simulink model "Noa_Nofusion"  (R2020b)
settings: Solver=FixedStepDiscrete  StartTime=0.0  StopTime=Inf  FixedStep=0.01  RelTol=1e-3
PostLoadFcn:
  | if any(exist('dsrtsu_mdlpostloadfcn', 'file') ~= 0), dsrtsu_mdlpostloadfcn('Execute', bdroot); end
InitFcn:
  | , if any(exist('rtifpga_mdlclblib', 'file') ~= 0), rtifpga_mdlclblib('Init', bdroot); end,
  | , if any(exist('dsmpb_private', 'file') ~= 0), dsmpb_private('dsmpb_mdlclblib', 'Init', bdroot); end,
undefined symbols (not defined in the file or in its folder): ACC_TimeGap_DecSetSwt, ACC_TimeGap_IncSetSwt, AccelPedalPosn, AccelPedalPosnVldty, AccelPedlPosnDiagc, AccPedalOverride, ACU_ShiftInProgress, ADAS_Posn_CurLane, AESSwtReq, ALC_SwtReq, BrkPedalSts, CC_ACC_CANCEL_OFFSwt, CC_ACC_CRUISE_OFFSwt, CC_ACC_DecSetSpd_SetSwt, CC_ACC_IncSetSpd_ResuSwt, CC_ACCSwtErr, CharSpd_ms, CSA_NODE, CURRENT_GEAR, CurrentGearValid, DiscIntNeverNeededParam, DrvDoorSts, DrvSBR, DrvTrqReqOvld, ECMACCInterface, ECMRespACC, ELKSwtReq, EngLimpHomeSts, EngSpd, EngState, EngState_PHEV, EngTrqMaxActSpd, EngTrqMinAct, EPS_DrvInpTrqVal_HighReslolution, EPS_FailSts, EPS_LKATorqOvrlDlvd, EPS_LKATorqOvrlDlvdVld, EPS_LKATrqOvlDlvdSts, EPS_SteerMod, EPS_TrqSnsrSts, EQ4_APPINFO, EQ4_LA_ELEM, EQ4_LA_HDR, EQ4_LAP_ELEM, EQ4_LAP_HDR, EQ4_LH_ELEM, EQ4_LH_HDR, EQ4_LRE_ELEM, EQ4_LRE_HDR, ESS_PedSwtReq, ESS_VehSwtReq, FFogLmpSts_F_Pbox, FLWheelDriveDirection, FLWheelSpd, FrntWiprSwtSts, FrntWshrSwtSts, FRWheelDriveDirection, FRWheelSpd, HazardLmpSwtSts, HCU_AccelPedalPosn_Diag ... (+151)
libraries: simulink x144, dsmpblib x33, canfdmsglib x10
(part 19 of 20)

== matlab function Noa_Nofusion/TOS/Subsystem2/DOP/HWA_Task100ms1/Dyc ==
  data: kapTrajFiltK1 input single size=1; vRef input single size=1; kapTrajFilt output single size=1; kapCourseErr output single; kapTraj input single size=1; alpSideSlipAngle input single size=1; A2 input single size=1; A1 input single size=1; LineValid input boolean size=1; ObjDx input single size=15; ObjDy input single size=15; TarLineValid input boolean; TarLineA2 input single; TarLineA1 input single; TarLineA0 input single size=1; dxC0 output single size=1; aPC0 output single size=1; bPC0 output single size=1; cPC0 output single size=1; aPC1 output single size=1; bPC1 output single size=1; cPC1 output single size=1; ObjDyc output single size=15
function [kapTrajFilt,kapCourseErr,dxC0,aPC0,bPC0,cPC0,aPC1,bPC1,cPC1,ObjDyc] = ...
    DriveCourseCalc(kapTrajFiltK1,vRef,kapTraj,alpSideSlipAngle,...
    A2,A1,LineValid,ObjDx,ObjDy,TarLineValid,TarLineA2,TarLineA1,TarLineA0)

ObjDyc = single(zeros(15,1));

if vRef>8.33
    t_alpSideSlipAngle = -alpSideSlipAngle;
else
    t_alpSideSlipAngle = single(0);
end

temp1 = single(0.1)/(single(0.1) + interpolate(single(24),single(0),single(55),single(0.4),vRef));

kapTrajFilt = kapTrajFiltK1 + temp1*(kapTraj - kapTrajFiltK1);

temp1 = abs(kapTraj*vRef);

if (temp1<0.001)&&(vRef>8.3)
    t_kapTrajwHyst = single(0);
else
    t_kapTrajwHyst = kapTrajFilt;
end

if TarLineValid
    temp = interpolate(single(0.2),single(0.2),single(1.5),single(1),abs(TarLineA0));
    dxC0Min = single(3);
else
    temp = single(1);
    dxC0Min = single(10);
end

dxC0 = max(vRef*temp,dxC0Min);
aPC0 = 0.5*t_kapTrajwHyst*(single(1)+1.5*t_alpSideSlipAngle*t_alpSideSlipAngle);
bPC0 = t_alpSideSlipAngle;
cPC0 = single(0);

temp1 = single(0.1)*abs(t_kapTrajwHyst);
temp2 = min(single(0.00013),single(0.004)/max(vRef,single(10)));
kapCourseErr = max(temp1,temp2);

aPC1 = aPC0;
bPC1 = bPC0;
cPC1 = single(0);

Low = interpolate(single(4),single(1),single(20),single(0),abs(atan(A1)));    % low vehiclespeed lanechange Angle is 4deg~20deg;
High = interpolate(single(4),single(1),single(10),single(0),abs(atan(A1)));   % low vehiclespeed lanechange Angle is 4deg~10deg;
t_vRefFactor = interpolate(single(5),Low,single(25),High,vRef);

t_Factor = single(1)*t_vRefFactor;

if TarLineValid==true
    aPC1 = TarLineA2;
    bPC1 = TarLineA1;
    cPC1 = (aPC0 - aPC1)*dxC0*dxC0 + (bPC0 - bPC1)*dxC0;
else
    if LineValid
        aPC1 = aPC0*(1 - t_Factor) + A2*t_Factor;
        bPC1 = bPC0*(1 - t_Factor) + A1*t_Factor;
        cPC1 = (aPC0 - aPC1)*dxC0*dxC0 + (bPC0 - bPC1)*dxC0;
    end
end

for i=1:15
   if ObjDx(i)>dxC0
      ObjDyc(i) =  ObjDy(i) - (aPC1*ObjDx(i)*ObjDx(i) + bPC1*ObjDx(i) + cPC1);
   else
      ObjDyc(i) =  ObjDy(i) - (aPC0*ObjDx(i)*ObjDx(i) + bPC0*ObjDx(i));
   end
end
end


function out = interpolate(x1,z1,x2,z2,Raw)
if Raw<=x1
    out = z1;
else
    if Raw>=x2
        out = z2;
    else
        out = z1 + (Raw-x1)*(z2-z1)/(x2-x1);
    end
end
end

== matlab function Noa_Nofusion/CR_RSDS_Input/MATLAB Function1 ==
  data: ObjNumber input uint8 size=1; ObjPrio output single size=24; ObjID input uint8 size=24; ObjDx input single size=24; ObjMatrix output single size=24
function [ObjPrio,ObjMatrix] = fcn(ObjNumber,ObjID,ObjDx)
%#codegen
ObjPrio = single(zeros(24,1));

for i=1:ObjNumber
    if ObjID(i)>0
        ObjPrio(i)=single(255) - abs(ObjDx(i));
    else
        ObjPrio(i)=single(0);
    end
end

ObjMatrix=ObjPrio;

t_h=1;
while 1
    t_h = t_h*3+1;
    if t_h>=ObjNumber
        break;
    end
end

%   t_h = 121;
while 1
    t_h = fix(t_h/3);
    for i=(t_h+1):ObjNumber
        j=i;
        t_zw=ObjMatrix(i);
        while (j>t_h)&&(t_zw<ObjMatrix(j-t_h))
            ObjMatrix(j)=ObjMatrix(j-t_h);
            j=j-t_h;
        end
        ObjMatrix(j)=t_zw;
    end
    if t_h==1
        break;
    end
end
end

== matlab function Noa_Nofusion/CR_RSDS_Input/MATLAB Function2 ==
  data: Prio input single size=24; Matrix input single size=24; ID input uint8 size=24; ObjID output uint8 size=11; Dx input single size=24; Dy input single size=24; ObjDx output single size=11; Vx input single size=24; Vy input single size=24; Ax input single size=24; Age input uint8 size=24; MoveSts input uint8 size=24; ObjDy output single size=11; ObjVx output single size=11; ObjVy output single size=11; ObjAx output single size=11; ObjAge output uint8 size=11; ObjMoveSts output uint8 size=11; FusType input uint8 size=24; ObjFusType output uint8 size=11
function [ObjID,ObjDx,ObjDy,ObjVx,ObjVy,ObjAx,ObjAge,ObjMoveSts,ObjFusType] =...
    fcn(Prio,Matrix,ID,Dx,Dy,Vx,Vy,Ax,Age,MoveSts,FusType)
%#codegen
ObjPrioLimit = Matrix(24-11);
ObjID = uint8(zeros(11,1));
ObjDx = single(zeros(11,1));
ObjDy = single(zeros(11,1));
ObjVx = single(zeros(11,1));
ObjVy = single(zeros(11,1));
ObjAx = single(zeros(11,1));
ObjAge = uint8(zeros(11,1));
ObjMoveSts = uint8(zeros(11,1));
ObjFusType = uint8(zeros(11,1));
Num = uint8(0);

for i=1:24
  if ID(i)>0 && Prio(i)>ObjPrioLimit
      Num = Num + uint8(1);
      ObjID(Num) = uint8(i);
      ObjDx(Num) = Dx(i);
      ObjDy(Num) = Dy(i);
      ObjVx(Num) = Vx(i);
      ObjVy(Num) = Vy(i);
      ObjAx(Num) = Ax(i);
      ObjAge(Num) = Age(i);
      ObjMoveSts(Num) = MoveSts(i);
      ObjFusType(Num) = FusType(i);
  end
end

== matlab function Noa_Nofusion/CR_RSDS_Input/RSDS_L_Bus/RSDS_L ==
  data: RadarID input uint8 size=1; ID input uint8 size=6; Dx input single size=6; Dy input single size=6; Vx input single size=6; Vy input single size=6; Ax input single size=6; ObjIDK1 input uint8 size=6; P output uint8 size=6; ObjDx output single size=6; ObjDy output single size=6; ObjVx output single size=6; ObjVy output single size=6; ObjAx output single size=6; ObjMoveSts output uint8 size=6; ObjFusType output uint8 size=6; ObjID output uint8 size=6; ObjAgeK1 input uint8 size=6; ObjAge output uint8 size=6
function [P,ObjDx,ObjDy,ObjVx,ObjVy,ObjAx,ObjMoveSts,ObjFusType,ObjID,ObjAge] =...
    DataT(RadarID,ID,Dx,Dy,Vx,Vy,Ax,ObjIDK1,ObjAgeK1)

if RadarID==uint8(1)
    FusFac = 4;
elseif RadarID==uint8(2)
    FusFac = 8;
elseif RadarID==uint8(3)
    FusFac = 16;
else
    FusFac = 32;
end

ObjID = uint8(zeros(6,1));
ObjDx = single(zeros(6,1));
ObjDy = single(zeros(6,1));
ObjVx = single(zeros(6,1));
ObjVy = single(zeros(6,1));
ObjAx = single(zeros(6,1));
ObjAge = uint8(ones(6,1));
ObjMoveSts = uint8(2*ones(6,1));
ObjFusType = uint8(FusFac*ones(6,1));

T = uint8(zeros(6,1));
P = uint8(zeros(6,1));
Index01 = uint8(zeros(6,1));
Index02 = uint8(zeros(6,1));
M = uint8(0);
N = uint8(0);
w = uint8(0);

for i=uint8(1):uint8(6)
    for j=uint8(1):uint8(6)
        if ID(i)==ObjIDK1(j) && ID(i)>uint8(0)
            T(j) = i;
            P(i) = j;
        end
    end
end

for j=uint8(1):uint8(6)
    if T(j)==uint8(0)
        if ObjIDK1(j)==uint8(0)
            N = N + uint8(1);
            Index01(N) = j;
        else
            M = M + uint8(1);
            Index02(M) = j;
        end
    end
end

for i=uint8(1):uint8(6)
    if P(i)==uint8(0) && ID(i)>uint8(0)
        w = w + uint8(1);
        if w<=N
            P(i) = Index01(w);
        else
            P(i) = Index02(w - N);
        end
    elseif P(i)>uint8(0)
        ObjAge(P(i)) = min(ObjAgeK1(i) + uint8(1),uint8(255));
    end
    if P(i)>uint8(0)
       ObjID(P(i)) = ID(i);
       ObjDx(P(i)) = Dx(i);
       ObjDy(P(i)) = Dy(i);
       ObjVx(P(i)) = Vx(i);
       ObjVy(P(i)) = Vy(i);
       ObjAx(P(i)) = Ax(i);
    end
end
for i=uint8(1):uint8(6)
    if ObjID(i)==uint8(0)
        ObjAge(i) = uint8(0);
        ObjMoveSts(i) = uint8(0);
        ObjFusType(i) = uint8(0);
    end
end
end

== matlab function Noa_Nofusion/CR_RSDS_Input/RSDS_R_Bus/RSDS_R ==
  data: RadarID input uint8 size=1; ID input uint8 size=6; Dx input single size=6; Dy input single size=6; Vx input single size=6; Vy input single size=6; Ax input single size=6; ObjIDK1 input uint8 size=6; P output uint8 size=6; ObjDx output single size=6; ObjDy output single size=6; ObjVx output single size=6; ObjVy output single size=6; ObjAx output single size=6; ObjMoveSts output uint8 size=6; ObjFusType output uint8 size=6; ObjID output uint8 size=6; ObjAgeK1 input uint8 size=6; ObjAge output uint8 size=6
function [P,ObjDx,ObjDy,ObjVx,ObjVy,ObjAx,ObjMoveSts,ObjFusType,ObjID,ObjAge] =...
    DataT(RadarID,ID,Dx,Dy,Vx,Vy,Ax,ObjIDK1,ObjAgeK1)

if RadarID==uint8(1)
    FusFac = 4;
elseif RadarID==uint8(2)
    FusFac = 8;
elseif RadarID==uint8(3)
    FusFac = 16;
else
    FusFac = 32;
end

ObjID = uint8(zeros(6,1));
ObjDx = single(zeros(6,1));
ObjDy = single(zeros(6,1));
ObjVx = single(zeros(6,1));
ObjVy = single(zeros(6,1));
ObjAx = single(zeros(6,1));
ObjAge = uint8(ones(6,1));
ObjMoveSts = uint8(2*ones(6,1));
ObjFusType = uint8(FusFac*ones(6,1));

T = uint8(zeros(6,1));
P = uint8(zeros(6,1));
Index01 = uint8(zeros(6,1));
Index02 = uint8(zeros(6,1));
M = uint8(0);
N = uint8(0);
w = uint8(0);

for i=uint8(1):uint8(6)
    for j=uint8(1):uint8(6)
        if ID(i)==ObjIDK1(j) && ID(i)>uint8(0)
            T(j) = i;
            P(i) = j;
        end
    end
end

for j=uint8(1):uint8(6)
    if T(j)==uint8(0)
        if ObjIDK1(j)==uint8(0)
            N = N + uint8(1);
            Index01(N) = j;
        else
            M = M + uint8(1);
            Index02(M) = j;
        end
    end
end

for i=uint8(1):uint8(6)
    if P(i)==uint8(0) && ID(i)>uint8(0)
        w = w + uint8(1);
        if w<=N
            P(i) = Index01(w);
        else
            P(i) = Index02(w - N);
        end
    elseif P(i)>uint8(0)
        ObjAge(P(i)) = min(ObjAgeK1(i) + uint8(1),uint8(255));
    end
    if P(i)>uint8(0)
       ObjID(P(i)) = ID(i);
       ObjDx(P(i)) = Dx(i);
       ObjDy(P(i)) = Dy(i);
       ObjVx(P(i)) = Vx(i);
       ObjVy(P(i)) = Vy(i);
       ObjAx(P(i)) = Ax(i);
    end
end
for i=uint8(1):uint8(6)
    if ObjID(i)==uint8(0)
        ObjAge(i) = uint8(0);
        ObjMoveSts(i) = uint8(0);
        ObjFusType(i) = uint8(0);
    end
end
end

== matlab function Noa_Nofusion/TOS/Subsystem2/DOP/HWA_Task100ms1/DycCutIn ==
  data: ObjValid input boolean size=15; ObjDyc input single size=15; ObjMoveSts input uint8 size=15; ObjDycCutIn output single size=15; ObjMove_b output boolean size=15; ObjCnt input uint8 size=15; ObjDycHist input single size=15; ObjqDycHist input single size=15; dycFiltK1 input single size=15; ObjDycFilt output single size=15
function [ObjDycCutIn,ObjMove_b,ObjDycFilt] = ...
    ObjDycCutInCalc(ObjValid,ObjDyc,ObjMoveSts,ObjCnt,ObjDycHist,ObjqDycHist,dycFiltK1)
 
ObjDycCutIn = single(zeros(15,1));
ObjDycFilt = single(zeros(15,1));
ObjMove_b = false(15,1); 
 
for i=1:15
    if ObjValid(i)
        t_dyc = ObjDyc(i);
        t_dycHist = ObjDycHist(i);
        t_qDycHist = ObjqDycHist(i);
        
        weightDycHist = t_qDycHist*0.1;
        weightDyc = single(1) - weightDycHist;
        
        t_dycASI = weightDycHist*t_dycHist + weightDyc*t_dyc;
        ObjDycCutIn(i) = t_dycASI;
        
        if ObjCnt(i)>2
            ObjDycFilt(i) = 0.028*(t_dycASI - dycFiltK1(i)) + dycFiltK1(i);
        else
            ObjDycFilt(i) = t_dycASI;
        end
        if ObjMoveSts(i)==2
            ObjMove_b(i) = true;
        end
    end
end

== matlab function Noa_Nofusion/SimBCM/BCMsim ==
  data: SimLeLmp input; CSASim_LampReq output; SimRiLmp input; Model_IDC_L2_LampReq input
function CSASim_LampReq = fcn(SimLeLmp, SimRiLmp, Model_IDC_L2_LampReq)
CSASim_LampReq=Model_IDC_L2_LampReq;
if SimRiLmp
    CSASim_LampReq=uint8(2);
end
if SimLeLmp
    CSASim_LampReq=uint8(1);
end

== matlab function Noa_Nofusion/TOS/Subsystem2/DOP/HWA_Task100ms1/DycHistCalc ==
  data: TrajHistBufferBTrajEnd input boolean; ObjTrajNumber input uint8; ObjDycHist output single; TrajCurrentIndex input uint8; TrajHistBufferBValid input boolean; TrajHistBufferDxv input single; TrajHistBufferDyv input single; ObjValid input boolean; ObjqDycHist output single; dxC0 input; aP0 input; bP0 input; cP0 input; aP1 input; bP1 input; cP1 input
function [ObjDycHist,ObjqDycHist] = DycHistCalc(TrajHistBufferBTrajEnd,ObjTrajNumber,TrajCurrentIndex,...
    TrajHistBufferBValid,TrajHistBufferDxv,TrajHistBufferDyv,ObjValid,dxC0,aP0,bP0,cP0,aP1,bP1,cP1)

t_dxv = single(0);
t_dyv = single(0);
t_dxvK1 = single(0);
t_dyvK1 = single(0);
ObjDycHist = single(zeros(15,1));
ObjqDycHist = single(zeros(15,1));

for iObj=1:15
    t_TrajNumber = ObjTrajNumber(iObj);
    if t_TrajNumber<21
        t_End = false;
        t_Failed = false;
        t_TrajCurrentIndex = TrajCurrentIndex(t_TrajNumber);
        t_TrajEnd = TrajHistBufferBTrajEnd(t_TrajNumber,t_TrajCurrentIndex);
        if (ObjValid(iObj)==true)&&(t_TrajEnd==false)
            for k=1:24
                if t_End==false
                    if t_TrajCurrentIndex<k
                        t_Index = t_TrajCurrentIndex + uint8(25) - k;
                    else
                        t_Index = t_TrajCurrentIndex - k + uint8(1);
                    end
                    if t_Index==1
                        t_IndexK1 = uint8(24);
                    else
                        t_IndexK1 = t_Index - uint8(1);
                    end
                    t_ValidK1 = TrajHistBufferBValid(t_TrajNumber,t_IndexK1);
                    t_TrajEndK1 = TrajHistBufferBTrajEnd(t_TrajNumber,t_IndexK1);
                    t_dxv = TrajHistBufferDxv(t_TrajNumber,t_Index);
                    t_dxvK1 = TrajHistBufferDxv(t_TrajNumber,t_IndexK1);
                    t_dyv = TrajHistBufferDyv(t_TrajNumber,t_Index);
                    t_dyvK1 = TrajHistBufferDyv(t_TrajNumber,t_IndexK1);
                    
                    if (t_TrajEndK1==true)||(t_ValidK1==false)
                        t_End = true;
                        t_Failed = true;
                    end
                    if (t_dxv>=0)&&(t_dxvK1<=0)
                        t_End = true;
                    end
                end
            end
        end
        if (t_End==true)&&(t_Failed==false)
            if (t_dxv==t_dxvK1)
                t_dycHist = t_dyv;
            else
                t_dycHist = t_dyv - t_dxv*(t_dyvK1 - t_dyv)/(t_dxvK1 - t_dxv);
            end
            t_qDycHist = single(1);  
        else
            if (t_End==true)&&(t_Failed==true)&&(t_dxv>0)
                if t_dxv>(dxC0)
                    t_dycHist = t_dyv - (aP1*t_dxv*t_dxv + bP1*t_dxv + cP1); 
                else
                    t_dycHist = t_dyv - (aP0*t_dxv*t_dxv + bP0*t_dxv + cP0); 
                end
               t_qDycHist = max((single(80) - t_dxv)/single(80),single(0));
            else
                t_dycHist = single(0);
                t_qDycHist = single(0);
            end
        end
    else
        t_dycHist = single(0);
        t_qDycHist = single(0);
    end
    ObjDycHist(iObj) = t_dycHist;
    ObjqDycHist(iObj) = t_qDycHist;
end

== stateflow chart Noa_Nofusion/SimBCM/CSALampCtrlSim/Chart1 ==
  state OFF
    en:
    SwtSts=false;
  state Hold
    en:
    SwtSts=true;
  state LeCloseReady
  (default) -> OFF
  LeCloseReady -> OFF : [SteerWheelAng<P_LmpCloseAngClose...
      | ||OFF]
  Hold -> OFF [order 2] : [OFF]
  OFF -> Hold : [ON]
  Hold -> LeCloseReady [order 1] : [SteerWheelAng>P_LmpCloseAngReady]
  data: SwtSts output; OFF input; ON input; SteerWheelAng input; P_LmpCloseAngClose input; P_LmpCloseAngReady input

== matlab function Noa_Nofusion/Subsystem4/LHLine ==
  data: LH_Count input; LH1A0 input single size=1; LH1A1 input single size=1; LH1A2 input single size=1; LH1A3 input single size=1; LH1RaMin input single size=1; LH1RaMax input single size=1; LH1Conf output uint8 size=1; LH1Avail input uint8 size=1; LH1LineType input uint8 size=1; LH1DLType input uint8 size=1; LH1SideType input uint8 size=1; LH1Wid input single size=1; LH1Crossing input; LH1Confidence input; LH2A0 input single size=1; LH2A1 input single size=1; LH2A2 input single size=1; LH2A3 input single size=1; LH2RaMin input single size=1; LH2RaMax input single size=1; LH2Avail input uint8 size=1; LH2LineType input uint8 size=1; LH2DLType input uint8 size=1; LH2SideType input uint8 size=1; LH2Wid input single size=1; LH1C0 output single size=1; LH1C1 output single size=1; LH1C2 output single size=1; LH1C3 output single size=1; LH1DxMin output single size=1; LH1DxMax output single size=1; LH1Type output uint8 size=1; LH1DLM output uint8 size=1; LH1Width output single size=1; LH1Reliable output; LeftLaneChange output uint8 size=1; LH2Conf output uint8 size=1; LH2C0 output single size=1; LH2C1 output single size=1; LH2C2 output single size=1; LH2C3 output single size=1; LH2DxMin output single size=1; LH2DxMax output single size=1; LH2Type output uint8 size=1; LH2DLM output uint8 size=1; LH2Width output single size=1; LH2Reliable output; RightLaneChange output uint8 size=1; LH2Crossing input; LH2Confidence input
function [LH1Conf,LH1C0,LH1C1,LH1C2,LH1C3,LH1DxMin,LH1DxMax,LH1Type,LH1DLM,LH1Width,LH1Reliable,LeftLaneChange,...
    LH2Conf,LH2C0,LH2C1,LH2C2,LH2C3,LH2DxMin,LH2DxMax,LH2Type,LH2DLM,LH2Width,LH2Reliable,RightLaneChange]...
    = LH(LH_Count,LH1A0,LH1A1,LH1A2,LH1A3,LH1RaMin,LH1RaMax,LH1Avail,LH1LineType,LH1DLType,LH1SideType,LH1Wid,LH1Crossing,LH1Confidence,...
    LH2A0,LH2A1,LH2A2,LH2A3,LH2RaMin,LH2RaMax,LH2Avail,LH2LineType,LH2DLType,LH2SideType,LH2Wid,LH2Crossing,LH2Confidence)

LH1Conf = uint8(0);
LH1C0 = single(0);
LH1C1 = single(0);
LH1C2 = single(0);
LH1C3 = single(0);
LH1DxMin = single(0);
LH1DxMax = single(0);
LH1Type = uint8(0);
LH1DLM = uint8(0);
LH1Width = single(0);
LH1Reliable = single(0);
LeftLaneChange = uint8(0);

LH2Conf = uint8(0);
LH2C0 = single(0);
LH2C1 = single(0);
LH2C2 = single(0);
LH2C3 = single(0);
LH2DxMin = single(0);
LH2DxMax = single(0);
LH2Type = uint8(0);
LH2DLM = uint8(0);
LH2Width = single(0);
LH2Reliable = single(0);
RightLaneChange = uint8(0);


%%
if LH_Count >= 1
    if LH1SideType==1
        LH1Conf = LH1Avail;
        LH1C0 = LH1A0;
        LH1C1 = LH1A1;
        LH1C2 = LH1A2;
        LH1C3 = LH1A3;
        LH1DxMin = LH1RaMin;
        LH1DxMax = LH1RaMax;
        LH1Type = LH1LineType;
        LH1DLM = LH1DLType;
        LH1Width = LH1Wid;
        LH1Reliable = LH1Confidence;
        LeftLaneChange = LH1Crossing;
    elseif LH1SideType==2
        LH2Conf = LH1Avail;
        LH2C0 = LH1A0;
        LH2C1 = LH1A1;
        LH2C2 = LH1A2;
        LH2C3 = LH1A3;
        LH2DxMin = LH1RaMin;
        LH2DxMax = LH1RaMax;
        LH2Type = LH1LineType;
        LH2DLM = LH1DLType;
        LH2Width = LH1Wid;
        LH2Reliable = LH1Confidence;
        RightLaneChange = LH1Crossing;
    end
    if LH_Count >= 2
        if LH2SideType==1
            LH1Conf = LH2Avail;
            LH1C0 = LH2A0;
            LH1C1 = LH2A1;
            LH1C2 = LH2A2;
            LH1C3 = LH2A3;
            LH1DxMin = LH2RaMin;
            LH1DxMax = LH2RaMax;
            LH1Type = LH2LineType;
            LH1DLM = LH2DLType;
            LH1Width = LH2Wid;
            LH1Reliable = LH2Confidence;
            LeftLaneChange = LH2Crossing;
        elseif LH2SideType==2
            LH2Conf = LH2Avail;
            LH2C0 = LH2A0;
            LH2C1 = LH2A1;
            LH2C2 = LH2A2;
            LH2C3 = LH2A3;
            LH2DxMin = LH2RaMin;
            LH2DxMax = LH2RaMax;
            LH2Type = LH2LineType;
            LH2DLM = LH2DLType;
            LH2Width = LH2Wid;
            LH2Reliable = LH2Confidence;
            RightLaneChange = LH2Crossing;
        end
    end
end

== matlab function Noa_Nofusion/Subsystem4/MATLAB Function5 ==
  data: IFV2RearAxis input single size=1; a0 output single size=1; a1 output single size=1; a2 output single size=1; a3 output single size=1; IFV2CenterAxis input single size=1; A0 input single size=1; A1 input single size=1; A2 input single size=1; A3 input single size=1; Range_min input single size=1; Rmin output single size=1; Range_max input single size=1; Rmax output single size=1
function [a0,a1,a2,a3,Rmin,Rmax] = ...
    fcn(IFV2RearAxis,IFV2CenterAxis,A0,A1,A2,A3,Range_min,Range_max)

Rmin = Range_min + IFV2RearAxis;
Rmax = Range_max + IFV2RearAxis;

if Range_max>0
   xi = [10;20;40;80];
   yi = -A3*xi.^3 - A2*xi.^2 - A1*xi - A0 + IFV2CenterAxis;
   xi = xi + IFV2RearAxis;
   [a3,a2,a1,a0] = pl(xi,yi);
else
    a3 = single(0);
    a2 = single(0);
    a1 = single(0);
    a0 = single(0);
end

== matlab function Noa_Nofusion/Subsystem4/MATLAB Function6 ==
  data: IFV2RearAxis input single size=1; a0 output single size=1; a1 output single size=1; a2 output single size=1; a3 output single size=1; IFV2CenterAxis input single size=1; A0 input single size=1; A1 input single size=1; A2 input single size=1; A3 input single size=1; Range_min input single size=1; Rmin output single size=1; Range_max input single size=1; Rmax output single size=1
function [a0,a1,a2,a3,Rmin,Rmax] = ...
    fcn(IFV2RearAxis,IFV2CenterAxis,A0,A1,A2,A3,Range_min,Range_max)

Rmin = Range_min + IFV2RearAxis;
Rmax = Range_max + IFV2RearAxis;

if Range_max>0
   xi = [10;20;40;80];
   yi = -A3*xi.^3 - A2*xi.^2 - A1*xi - A0 + IFV2CenterAxis;
   xi = xi + IFV2RearAxis;
   [a3,a2,a1,a0] = pl(xi,yi);
else
    a3 = single(0);
    a2 = single(0);
    a1 = single(0);
    a0 = single(0);
end

== matlab function Noa_Nofusion/Subsystem4/Simulink Function/MATLAB Function3 ==
  data: IFV2RearAxis input single size=1; a0 output single size=1; a1 output single size=1; a2 output single size=1; a3 output single size=1; IFV2CenterAxis input single size=1; A0 input single size=1; A1 input single size=1; A2 input single size=1; A3 input single size=1; Range_min input single size=1; Rmin output single size=1; Range_max input single size=1; Rmax output single size=1
function [a0,a1,a2,a3,Rmin,Rmax] = ...
    fcn(IFV2RearAxis,IFV2CenterAxis,A0,A1,A2,A3,Range_min,Range_max)

Rmin = Range_min + IFV2RearAxis;
Rmax = Range_max + IFV2RearAxis;

if Range_max>0
   xi = [10;20;40;80];
   yi = -A3*xi.^3 - A2*xi.^2 - A1*xi - A0 + IFV2CenterAxis;
   xi = xi + IFV2RearAxis;
   [a3,a2,a1,a0] = pl(xi,yi);
else
    a3 = single(0);
    a2 = single(0);
    a1 = single(0);
    a0 = single(0);
end

== stateflow chart Noa_Nofusion/SimBCM/CSALampCtrlSim/Chart2 ==
  state OFF
    en:
    SwtSts=false;
  state Hold
    en:
    SwtSts=true;
  state LeCloseReady
  (default) -> OFF
  LeCloseReady -> OFF : [abs(SteerWheelAng)>-P_LmpCloseAngClose...
      | ||OFF]
  Hold -> OFF [order 2] : [OFF]
  OFF -> Hold : [ON]
  Hold -> LeCloseReady [order 1] : [SteerWheelAng<-P_LmpCloseAngReady]
  data: SwtSts output; OFF input; ON input; SteerWheelAng input; P_LmpCloseAngClose input; P_LmpCloseAngReady input

== matlab function Noa_Nofusion/TOS/Subsystem2/DOP/HWA_Task100ms1/LostTargetCalc ==
  data: ObjValid input boolean size=15; ReID output uint8 size=1; ObjDx input single size=15; ObjDy input single size=15; DeltaDx input single size=1; DeltaDy input single size=1; P0IDK1 input uint8 size=1; P0VxK1 input single size=1; P0DxK1 input single size=1; P0DyK1 input single size=1; P0RangeK1 input; P0ArGK1 input; P0DycK1 input single size=1; P0VycK1 input single size=1; P0CutIn_bK1 input boolean size=1; tTargetLostK1 input single size=1; ReRange output single size=1; ReArG output single size=1; ReDx output single size=1; ReDy output single size=1; ReVx output single size=1; ReCutIn_b output boolean size=1; ReDyc output single size=1; ReVyc output single size=1; TargetLost_b output boolean size=1; Covered_b output boolean size=1; tTargetLost output single size=1
function [ReID,ReRange,ReArG,ReDx,ReDy,ReVx,ReCutIn_b,ReDyc,ReVyc,TargetLost_b,Covered_b,tTargetLost]...
    = LostTargetCalc(ObjValid,ObjDx,ObjDy,DeltaDx,DeltaDy,...
    P0IDK1,P0VxK1,P0DxK1,P0DyK1,P0RangeK1,P0ArGK1,P0DycK1,P0VycK1,P0CutIn_bK1,tTargetLostK1)
 
ReID = P0IDK1;
ReRange = single(255);
ReArG = single(0);
ReDx = single(255);
ReDy = single(0);
ReVx = single(0);
ReDyc = single(0);
ReVyc = single(0);
ReCutIn_b = false;
TargetLost_b = false;
tTargetLost = single(0);
Covered_b = false;
 
if (P0IDK1>0)&&(P0IDK1<100)    % k1 Exist Target
    if ObjValid(P0IDK1)==false
        ExistNearObj = false;
        P0DxPred = P0DxK1 + 0.1*P0VxK1;
        P0DyPred = P0DyK1;
        P0RangePred = P0RangeK1 + 0.1*P0VxK1; 
        for i=1:15
            if (ObjValid(i)==true)&&(ObjDx(i)<P0DxPred)
                Covered_b = CoveredCalc(P0DxPred,P0DyPred,ObjDx(i),ObjDy(i),single(2.1),single(-0.1));
                if Covered_b==true
                   break; 
                end
            end
            if (ObjValid(i)==1)&&(abs(ObjDx(i)-P0DxPred)<DeltaDx)&&(abs(ObjDy(i)-P0DyPred)<DeltaDy)
               ExistNearObj = true;
               ReID = uint8(i);
               ReDx = ObjDx(i);
            end
        end
        if (ExistNearObj==false)&&(Covered_b==false)
            TargetLost_b = true;
            tTargetLost = single(0.1);
            ReID = uint8(255);
            ReRange = P0RangePred;
            ReArG = P0ArGK1;
            ReDx = P0DxPred;
            ReDy = P0DyPred;
            ReVx = P0VxK1;
            ReCutIn_b = P0CutIn_bK1;
            ReVyc = P0VycK1;
            ReDyc = P0DycK1 + 0.1*P0VycK1;
        end
    end
else
    if P0IDK1>100   %  k1 Exist Target Re
        ExistNearObj = false;
        P0DxPred = P0DxK1 + 0.1*P0VxK1;
        P0DyPred = P0DyK1;
        P0RangePred = P0RangeK1 + 0.1*P0VxK1; 

        for i=1:15
            if (ObjValid(i)==1)&&(abs(ObjDx(i)-P0DxPred)<DeltaDx)&&(abs(ObjDy(i)-P0DyPred)<DeltaDy)
                ExistNearObj = true;
                ReID = uint8(i);
                ReDx = ObjDx(i);
                TargetLost_b = false;
                tTargetLost = single(0);
            end
        end
        if ExistNearObj==false
            TargetLost_b = true;
            tTargetLost = tTargetLostK1 + single(0.1);
            ReID = uint8(255);
            ReRange = P0RangePred;
            ReArG = P0ArGK1;
            ReDx = P0DxPred;
            ReDy = P0DyPred;
            ReVx = P0VxK1;
            ReCutIn_b = P0CutIn_bK1;
            ReVyc = P0VycK1;
            ReDyc = P0DycK1 + 0.1*P0VycK1;
        end
    end
end
end
 
function t_Covered_b = CoveredCalc(DxPred,DyPred,Dx,Dy,IFVDx,IFVDy)
y = (IFVDy - DyPred)*(Dx - DxPred)/(IFVDx - DxPred) + DyPred ;
Delta = single(0.8) + (Dx - IFVDx)/(DxPred - IFVDx);
if abs(Dy - y)<=Delta
    t_Covered_b = true;
else
    t_Covered_b = false;
end
end

== matlab function Noa_Nofusion/Subsystem4/LALine ==
  data: LA_Count input; L1Conf output uint8 size=1; L1C0 output single size=1; L1C1 output single size=1; L1C2 output single size=1; L1C3 output single size=1; L1DxMin output single size=1; L1DxMax output single size=1; L1A0 input single size=1; L1A1 input single size=1; L1A2 input single size=1; L1A3 input single size=1; L1RaMin input single size=1; L1RaMax input single size=1; L1Avail input uint8 size=1; L1LineType input uint8 size=1; L1DLType input uint8 size=1; L1SideType input uint8 size=1; L1Wid input single size=1; L1Confidence input; L2A0 input single size=1; L2A1 input single size=1; L2A2 input single size=1; L2A3 input single size=1; L2RaMin input single size=1; L2RaMax input single size=1; L2Avail input uint8 size=1; L2LineType input uint8 size=1; L2DLType input uint8 size=1; L2SideType input uint8 size=1; L2Wid input single size=1; L2Confidence input; L3A0 input single size=1; L3A1 input single size=1; L3A2 input single size=1; L3A3 input single size=1; L3RaMin input single size=1; L3RaMax input single size=1; L3Avail input uint8 size=1; L3LineType input uint8 size=1; L3DLType input uint8 size=1; L3SideType input uint8 size=1; L3Wid input single size=1; L3Confidence input; L4A0 input single size=1; L4A1 input single size=1; L4A2 input single size=1; L4A3 input single size=1; L4RaMin input single size=1; L4RaMax input single size=1; L4Avail input uint8 size=1; L4LineType input uint8 size=1; L4DLType input uint8 size=1; L4SideType input uint8 size=1; L4Wid input single size=1; L1Type output uint8 size=1; L1DLM output uint8 size=1; L1Width output single size=1; L1Reliable output; L2Conf output uint8 size=1; L2C0 output single size=1; L2C1 output single size=1; L2C2 output single size=1; L2C3 output single size=1; L2DxMin output single size=1; L2DxMax output single size=1; L2Type output uint8 size=1; L2DLM output uint8 size=1; L2Width output single size=1; L2Reliable output; L3Conf output uint8 size=1; L3C0 output single size=1; L3C1 output single size=1; L3C2 output single size=1; L3C3 output single size=1; L3DxMin output single size=1; L3DxMax output single size=1; L3Type output uint8 size=1; L3DLM output uint8 size=1; L3Width output single size=1; L3Reliable output; L4Conf output uint8 size=1; L4C0 output single size=1; L4C1 output single size=1; L4C2 output single size=1; L4C3 output single size=1; L4DxMin output single size=1; L4DxMax output single size=1; L4Type output uint8 size=1; L4DLM output uint8 size=1; L4Width output single size=1; L4Confidence input; L4Reliable output
function [L1Conf,L1C0,L1C1,L1C2,L1C3,L1DxMin,L1DxMax,L1Type,L1DLM,L1Width,L1Reliable,...
    L2Conf,L2C0,L2C1,L2C2,L2C3,L2DxMin,L2DxMax,L2Type,L2DLM,L2Width,L2Reliable,...
    L3Conf,L3C0,L3C1,L3C2,L3C3,L3DxMin,L3DxMax,L3Type,L3DLM,L3Width,L3Reliable,...
    L4Conf,L4C0,L4C1,L4C2,L4C3,L4DxMin,L4DxMax,L4Type,L4DLM,L4Width,L4Reliable]...
    = LA(LA_Count,L1A0,L1A1,L1A2,L1A3,L1RaMin,L1RaMax,L1Avail,L1LineType,L1DLType,L1SideType,L1Wid,L1Confidence,...
    L2A0,L2A1,L2A2,L2A3,L2RaMin,L2RaMax,L2Avail,L2LineType,L2DLType,L2SideType,L2Wid,L2Confidence,...
    L3A0,L3A1,L3A2,L3A3,L3RaMin,L3RaMax,L3Avail,L3LineType,L3DLType,L3SideType,L3Wid,L3Confidence,...
    L4A0,L4A1,L4A2,L4A3,L4RaMin,L4RaMax,L4Avail,L4LineType,L4DLType,L4SideType,L4Wid,L4Confidence)

L1Conf = uint8(0);
L1C0 = single(0);
L1C1 = single(0);
L1C2 = single(0);
L1C3 = single(0);
L1DxMin = single(0);
L1DxMax = single(0);
L1Type = uint8(0);
L1DLM = uint8(0);
L1Width = single(0);
L1Reliable = single(0);

L2Conf = uint8(0);
L2C0 = single(0);
L2C1 = single(0);
L2C2 = single(0);
L2C3 = single(0);
L2DxMin = single(0);
L2DxMax = single(0);
L2Type = uint8(0);
L2DLM = uint8(0);
L2Width = single(0);
L2Reliable = single(0);

L3Conf = uint8(0);
L3C0 = single(0);
L3C1 = single(0);
L3C2 = single(0);
L3C3 = single(0);
L3DxMin = single(0);
L3DxMax = single(0);
L3Type = uint8(0);
L3DLM = uint8(0);
L3Width = single(0);
L3Reliable = single(0);

L4Conf = uint8(0);
L4C0 = single(0);
L4C1 = single(0);
L4C2 = single(0);
L4C3 = single(0);
L4DxMin = single(0);
L4DxMax = single(0);
L4Type = uint8(0);
L4DLM = uint8(0);
L4Width = single(0);
L4Reliable = single(0);
%%  临车道车道线预处理
if LA_Count >= 1                                     %临车道车道线数量
    if L1SideType==1                                 %左左车道线
        L1Conf = L1Avail;
        L1C0 = L1A0;
        L1C1 = L1A1;
        L1C2 = L1A2;
        L1C3 = L1A3;
        L1DxMin = L1RaMin;
        L1DxMax = L1RaMax;
        L1Type = L1LineType;
        L1DLM = L1DLType;
        L1Width = L1Wid;
        L1Reliable = L1Confidence;
    elseif L1SideType==2                             %左车道右侧车道线
        L2Conf = L1Avail;
        L2C0 = L1A0;
        L2C1 = L1A1;
        L2C2 = L1A2;
        L2C3 = L1A3;
        L2DxMin = L1RaMin;
        L2DxMax = L1RaMax;
        L2Type = L1LineType;
        L2DLM = L1DLType;
        L2Width = L1Wid;
        L2Reliable = L1Confidence;
    elseif L1SideType==3                             %右车道左侧车道线
        L3Conf = L1Avail;
        L3C0 = L1A0;
        L3C1 = L1A1;
        L3C2 = L1A2;
        L3C3 = L1A3;
        L3DxMin = L1RaMin;
        L3DxMax = L1RaMax;
        L3Type = L1LineType;
        L3DLM = L1DLType;
        L3Width = L1Wid;
        L3Reliable = L1Confidence;
    elseif L1SideType==4                             %右右车道线
        L4Conf = L1Avail;
        L4C0 = L1A0;
        L4C1 = L1A1;
        L4C2 = L1A2;
        L4C3 = L1A3;
        L4DxMin = L1RaMin;
        L4DxMax = L1RaMax;
        L4Type = L1LineType;
        L4DLM = L1DLType;
        L4Width = L1Wid;
        L4Reliable = L1Confidence;
    end
    if LA_Count >= 2
        if L2SideType==1
            L1Conf = L2Avail;
            L1C0 = L2A0;
            L1C1 = L2A1;
            L1C2 = L2A2;
            L1C3 = L2A3;
            L1DxMin = L2RaMin;
            L1DxMax = L2RaMax;
            L1Type = L2LineType;
            L1DLM = L2DLType;
            L1Width = L2Wid;
            L1Reliable = L2Confidence;
        elseif L2SideType==2
            L2Conf = L2Avail;
            L2C0 = L2A0;
            L2C1 = L2A1;
            L2C2 = L2A2;
            L2C3 = L2A3;
            L2DxMin = L2RaMin;
            L2DxMax = L2RaMax;
            L2Type = L2LineType;
            L2DLM = L2DLType;
            L2Width = L2Wid;
            L2Reliable = L2Confidence;
        elseif L2SideType==3
            L3Conf = L2Avail;
            L3C0 = L2A0;
            L3C1 = L2A1;
            L3C2 = L2A2;
            L3C3 = L2A3;
            L3DxMin = L2RaMin;
            L3DxMax = L2RaMax;
            L3Type = L2LineType;
            L3DLM = L2DLType;
            L3Width = L2Wid;
            L3Reliable = L2Confidence;
        elseif L2SideType==4
            L4Conf = L2Avail;
            L4C0 = L2A0;
            L4C1 = L2A1;
            L4C2 = L2A2;
            L4C3 = L2A3;
            L4DxMin = L2RaMin;
            L4DxMax = L2RaMax;
            L4Type = L2LineType;
            L4DLM = L2DLType;
            L4Width = L2Wid;
            L4Reliable = L2Confidence;
        end
        if LA_Count >= 3
            if L3SideType==1
                L1Conf = L3Avail;
                L1C0 = L3A0;
                L1C1 = L3A1;
                L1C2 = L3A2;
                L1C3 = L3A3;
                L1DxMin = L3RaMin;
                L1DxMax = L3RaMax;
                L1Type = L3LineType;
                L1DLM = L3DLType;
                L1Width = L3Wid;
                L1Reliable = L3Confidence;
            elseif L3SideType==2
                L2Conf = L3Avail;
                L2C0 = L3A0;
                L2C1 = L3A1;
                L2C2 = L3A2;
                L2C3 = L3A3;
                L2DxMin = L3RaMin;
                L2DxMax = L3RaMax;
                L2Type = L3LineType;
                L2DLM = L3DLType;
                L2Width = L3Wid;
                L2Reliable = L3Confidence;
            elseif L3SideType==3
                L3Conf = L3Avail;
                L3C0 = L3A0;
                L3C1 = L3A1;
                L3C2 = L3A2;
                L3C3 = L3A3;
                L3DxMin = L3RaMin;
                L3DxMax = L3RaMax;
                L3Type = L3LineType;
                L3DLM = L3DLType;
                L3Width = L3Wid;
                L3Reliable = L3Confidence;
            elseif L3SideType==4
                L4Conf = L3Avail;
                L4C0 = L3A0;
                L4C1 = L3A1;
                L4C2 = L3A2;
                L4C3 = L3A3;
                L4DxMin = L3RaMin;
                L4DxMax = L3RaMax;
                L4Type = L3LineType;
                L4DLM = L3DLType;
                L4Width = L3Wid;
                L4Reliable = L3Confidence;
            end
            if LA_Count >= 4
                if L4SideType==1
                    L1Conf = L4Avail;
                    L1C0 = L4A0;
                    L1C1 = L4A1;
                    L1C2 = L4A2;
                    L1C3 = L4A3;
                    L1DxMin = L4RaMin;
                    L1DxMax = L4RaMax;
                    L1Type = L4LineType;
                    L1DLM = L4DLType;
                    L1Width = L4Wid;
                    L1Reliable = L4Confidence;
                elseif L4SideType==2
                    L2Conf = L4Avail;
                    L2C0 = L4A0;
                    L2C1 = L4A1;
                    L2C2 = L4A2;
                    L2C3 = L4A3;
                    L2DxMin = L4RaMin;
                    L2DxMax = L4RaMax;
                    L2Type = L4LineType;
                    L2DLM = L4DLType;
                    L2Width = L4Wid;
                    L2Reliable = L4Confidence;
                elseif L4SideType==3
                    L3Conf = L4Avail;
                    L3C0 = L4A0;
                    L3C1 = L4A1;
                    L3C2 = L4A2;
                    L3C3 = L4A3;
                    L3DxMin = L4RaMin;
                    L3DxMax = L4RaMax;
                    L3Type = L4LineType;
                    L3DLM = L4DLType;
                    L3Width = L4Wid;
                    L3Reliable = L4Confidence;
                elseif L4SideType==4
                    L4Conf = L4Avail;
                    L4C0 = L4A0;
                    L4C1 = L4A1;
                    L4C2 = L4A2;
                    L4C3 = L4A3;
                    L4DxMin = L4RaMin;
                    L4DxMax = L4RaMax;
                    L4Type = L4LineType;
                    L4DLM = L4DLType;
                    L4Width = L4Wid;
                    L4Reliable = L4Confidence;
                end
            end
        end
    end
end

== matlab function Noa_Nofusion/TOS/Subsystem2/DOP/HWA_Task100ms1/Lpb ==
  data: vRef input single size=1; alpSumSlideCurveness input single size=1; ObjValid input boolean size=15; ObjDyc input single size=15; ObjLpb output single size=15; ObjDycHist input single size=15; ObjqDycHist input single size=15; ObjLpbL output single size=15; ObjLpbR output single size=15; ObjVyc input single size=15; ObjYawAngle input single size=15; ObjDylaneEdgeRight input; ObjDyEdgeWidthRight input; ObjDylaneEdgeLeft input; ObjDyEdgeWidthLeft input
function [ObjLpb,ObjLpbL,ObjLpbR] = LpbCalc(vRef,alpSumSlideCurveness,...
    ObjValid,ObjDyc,ObjDycHist,ObjqDycHist,ObjVyc,ObjYawAngle,...
    ObjDylaneEdgeRight,ObjDyEdgeWidthRight,ObjDylaneEdgeLeft,ObjDyEdgeWidthLeft)

 [ObjLpb,ObjLpbL,ObjLpbR] = LpbCalc(vRef,alpSumSlideCurveness,...
    ObjValid,ObjDyc,ObjDycHist,ObjqDycHist,ObjVyc,ObjYawAngle,...
    ObjDylaneEdgeRight,ObjDyEdgeWidthRight,ObjDylaneEdgeLeft,ObjDyEdgeWidthLeft);
end

== matlab function Noa_Nofusion/TOS/Subsystem2/ACCOSM/HWA_Task100ms1/ACC_DisplayBar ==
  data: TimeGap input; DisplayBar output uint8; DesireDistance input; ACCmode input; TargetRange input; Scale input; TargetExist input; DisplayBarK1 input uint8
function DisplayBar = fcn(TimeGap,DesireDistance,ACCmode,TargetRange,Scale,TargetExist,DisplayBarK1)
%#codegen
DisplayBar = DisplayBarK1;

ScaleDis = Scale*DesireDistance;
upScaleDis = (Scale+single(0.05))*DesireDistance;
lowScaleDis = (Scale-single(0.05))*DesireDistance;

i = TimeGap;

if (ACCmode==0)||(ACCmode==7)
    DisplayBar = uint8(0);
else
    if TargetExist==false
        DisplayBar=uint8(0);
    else
        switch(DisplayBarK1)
            case uint8(0)
                 if TargetRange> ScaleDis(i,3)
                     DisplayBar=uint8(4);
                 else
                     if TargetRange>ScaleDis(i,2)
                         DisplayBar=uint8(3);
                     else
                         if TargetRange>ScaleDis(i,1)
                             DisplayBar=uint8(2);
                         else
                             DisplayBar=uint8(1);
                         end
                     end
                 end
            case uint8(1)
                 if TargetRange> upScaleDis(i,3)
                     DisplayBar=uint8(4);
                 else
                     if TargetRange>upScaleDis(i,2)
                         DisplayBar=uint8(3);
                     else
                         if TargetRange>upScaleDis(i,1)
                             DisplayBar=uint8(2);
                         else
                             DisplayBar=uint8(1);
                         end
                     end
                 end
            case uint8(2)
                 if TargetRange> upScaleDis(i,3)
                     DisplayBar=uint8(4);
                 else
                     if TargetRange>upScaleDis(i,2)
                         DisplayBar=uint8(3);
                     else
                         if TargetRange>lowScaleDis(i,1)
                             DisplayBar=uint8(2);
                         else
                             DisplayBar=uint8(1);
                         end
                     end
                 end   
            case uint8(3)
                 if TargetRange> upScaleDis(i,3)
                     DisplayBar=uint8(4);
                 else
                     if TargetRange>lowScaleDis(i,2)
                         DisplayBar=uint8(3);
                     else
                         if TargetRange>lowScaleDis(i,1)
                             DisplayBar=uint8(2);
                         else
                             DisplayBar=uint8(1);
                         end
                     end
                end
            case uint8(4)
                 if TargetRange> lowScaleDis(i,3)
                     DisplayBar=uint8(4);
                 else
                     if TargetRange>lowScaleDis(i,2)
                         DisplayBar=uint8(3);
                     else
                         if TargetRange>lowScaleDis(i,1)
                             DisplayBar=uint8(2);
                         else
                             DisplayBar=uint8(1);
                         end
                     end
                 end      
        end    
    end
end

== matlab function Noa_Nofusion/TOS/Subsystem2/ACCOSM/HWA_Task100ms1/Dyc ==
  data: kapTrajFiltK1 input single size=1; vRef input single size=1; kapTrajFilt output single size=1; kapCourseErr output single; kapTraj input single size=1; alpSideSlipAngle input single size=1; A2 input single size=1; A1 input single size=1; LineValid input boolean size=1; ObjDx input single size=15; ObjDy input single size=15; TarLineValid input boolean; TarLineA2 input single; TarLineA1 input single; TarLineA0 input single size=1; dxC0 output single size=1; aPC0 output single size=1; bPC0 output single size=1; cPC0 output single size=1; aPC1 output single size=1; bPC1 output single size=1; cPC1 output single size=1; ObjDyc output single size=15
function [kapTrajFilt,kapCourseErr,dxC0,aPC0,bPC0,cPC0,aPC1,bPC1,cPC1,ObjDyc] = ...
    DriveCourseCalc(kapTrajFiltK1,vRef,kapTraj,alpSideSlipAngle,...
    A2,A1,LineValid,ObjDx,ObjDy,TarLineValid,TarLineA2,TarLineA1,TarLineA0)

ObjDyc = single(zeros(15,1));

if vRef>8.33
    t_alpSideSlipAngle = -alpSideSlipAngle;
else
    t_alpSideSlipAngle = single(0);
end

temp1 = single(0.1)/(single(0.1) + interpolate(single(24),single(0),single(55),single(0.4),vRef));

kapTrajFilt = kapTrajFiltK1 + temp1*(kapTraj - kapTrajFiltK1);

temp1 = abs(kapTraj*vRef);

if (temp1<0.001)&&(vRef>8.3)
    t_kapTrajwHyst = single(0);
else
    t_kapTrajwHyst = kapTrajFilt;
end

if TarLineValid
    temp = interpolate(single(0.2),single(0.2),single(1.5),single(1),abs(TarLineA0));
    dxC0Min = single(3);
else
    temp = single(1);
    dxC0Min = single(10);
end

dxC0 = max(vRef*temp,dxC0Min);
aPC0 = 0.5*t_kapTrajwHyst*(single(1)+1.5*t_alpSideSlipAngle*t_alpSideSlipAngle);
bPC0 = t_alpSideSlipAngle;
cPC0 = single(0);

temp1 = single(0.1)*abs(t_kapTrajwHyst);
temp2 = min(single(0.00013),single(0.004)/max(vRef,single(10)));
kapCourseErr = max(temp1,temp2);

aPC1 = aPC0;
bPC1 = bPC0;
cPC1 = single(0);

Low = interpolate(single(4),single(1),single(20),single(0),abs(atan(A1)));    % low vehiclespeed lanechange Angle is 4deg~20deg;
High = interpolate(single(4),single(1),single(10),single(0),abs(atan(A1)));   % low vehiclespeed lanechange Angle is 4deg~10deg;
t_vRefFactor = interpolate(single(5),Low,single(25),High,vRef);

t_Factor = single(1)*t_vRefFactor;

if TarLineValid==true
    aPC1 = TarLineA2;
    bPC1 = TarLineA1;
    cPC1 = (aPC0 - aPC1)*dxC0*dxC0 + (bPC0 - bPC1)*dxC0;
else
    if LineValid
        aPC1 = aPC0*(1 - t_Factor) + A2*t_Factor;
        bPC1 = bPC0*(1 - t_Factor) + A1*t_Factor;
        cPC1 = (aPC0 - aPC1)*dxC0*dxC0 + (bPC0 - bPC1)*dxC0;
    end
end

for i=1:15
   if ObjDx(i)>dxC0
      ObjDyc(i) =  ObjDy(i) - (aPC1*ObjDx(i)*ObjDx(i) + bPC1*ObjDx(i) + cPC1);
   else
      ObjDyc(i) =  ObjDy(i) - (aPC0*ObjDx(i)*ObjDx(i) + bPC0*ObjDx(i));
   end
end
end


function out = interpolate(x1,z1,x2,z2,Raw)
if Raw<=x1
    out = z1;
else
    if Raw>=x2
        out = z2;
    else
        out = z1 + (Raw-x1)*(z2-z1)/(x2-x1);
    end
end
end

== matlab function Noa_Nofusion/TOS/Subsystem2/ACCOSM/HWA_Task100ms1/DycCutIn ==
  data: ObjValid input boolean size=15; ObjDyc input single size=15; ObjMoveSts input uint8 size=15; ObjDycCutIn output single size=15; ObjMove_b output boolean size=15; ObjCnt input uint8 size=15; ObjDycHist input single size=15; ObjqDycHist input single size=15; dycFiltK1 input single size=15; ObjDycFilt output single size=15
function [ObjDycCutIn,ObjMove_b,ObjDycFilt] = ...
    ObjDycCutInCalc(ObjValid,ObjDyc,ObjMoveSts,ObjCnt,ObjDycHist,ObjqDycHist,dycFiltK1)
 
ObjDycCutIn = single(zeros(15,1));
ObjDycFilt = single(zeros(15,1));
ObjMove_b = false(15,1); 
 
for i=1:15
    if ObjValid(i)
        t_dyc = ObjDyc(i);
        t_dycHist = ObjDycHist(i);
        t_qDycHist = ObjqDycHist(i);
        
        weightDycHist = t_qDycHist*0.1;
        weightDyc = single(1) - weightDycHist;
        
        t_dycASI = weightDycHist*t_dycHist + weightDyc*t_dyc;
        ObjDycCutIn(i) = t_dycASI;
        
        if ObjCnt(i)>2
            ObjDycFilt(i) = 0.028*(t_dycASI - dycFiltK1(i)) + dycFiltK1(i);
        else
            ObjDycFilt(i) = t_dycASI;
        end
        if ObjMoveSts(i)==2
            ObjMove_b(i) = true;
        end
    end
end
